simulink model "Ass_3_2024a"  (R2024a)
settings: Solver=VariableStepAuto  StartTime=0.0  StopTime=inf  RelTol=1e-3
model workspace (MAT data in the model file):
  SL_ROS_VariableLengthArrays_MaxSizes.CommonInfo.ArrayTruncateAction = 'EmitWarning'
  SL_ROS_VariableLengthArrays_MaxSizes.MsgTypeMap = containers.Map
  SL_ROS_VariableLengthArrays_MaxSizes.MsgTypeMap.serialization.keys = {'sensor_msgs/Image'}
  SL_ROS_VariableLengthArrays_MaxSizes.MsgTypeMap.serialization.values{1}(1).PropertyName = 'Data'
  SL_ROS_VariableLengthArrays_MaxSizes.MsgTypeMap.serialization.values{1}(1).DataType = 'uint8'
  SL_ROS_VariableLengthArrays_MaxSizes.MsgTypeMap.serialization.values{1}(1).MaxLength = 921600
  SL_ROS_VariableLengthArrays_MaxSizes.MsgTypeMap.serialization.values{1}(2).PropertyName = 'Encoding'
  SL_ROS_VariableLengthArrays_MaxSizes.MsgTypeMap.serialization.values{1}(2).DataType = 'uint8'
  SL_ROS_VariableLengthArrays_MaxSizes.MsgTypeMap.serialization.values{1}(2).MaxLength = 128
  SL_ROS_VariableLengthArrays_MaxSizes.MsgTypeMap.serialization.uniformity = 0
  SL_ROS_VariableLengthArrays_MaxSizes.MsgTypeMap.serialization.keyType = 'char'
  SL_ROS_VariableLengthArrays_MaxSizes.MsgTypeMap.serialization.valueType = 'any'
undefined symbols (not defined in the file or in its folder): Angular, gray, Linear, Rec, SDTV
libraries: robotlib x4, simulink x2, visionstatistics x1, visionconversions x1
settings Model: Creator=daniele

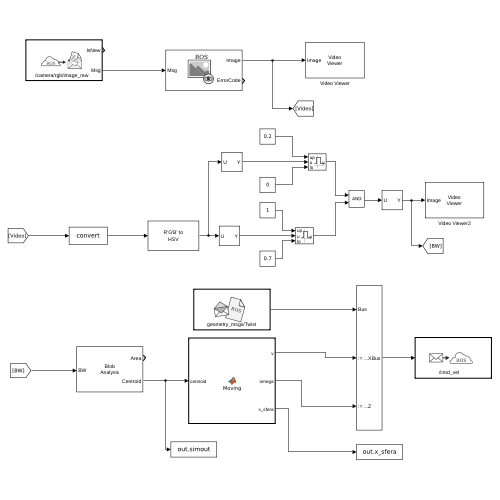
[thumbnail: Simulink's stored preview of the top-level diagram]
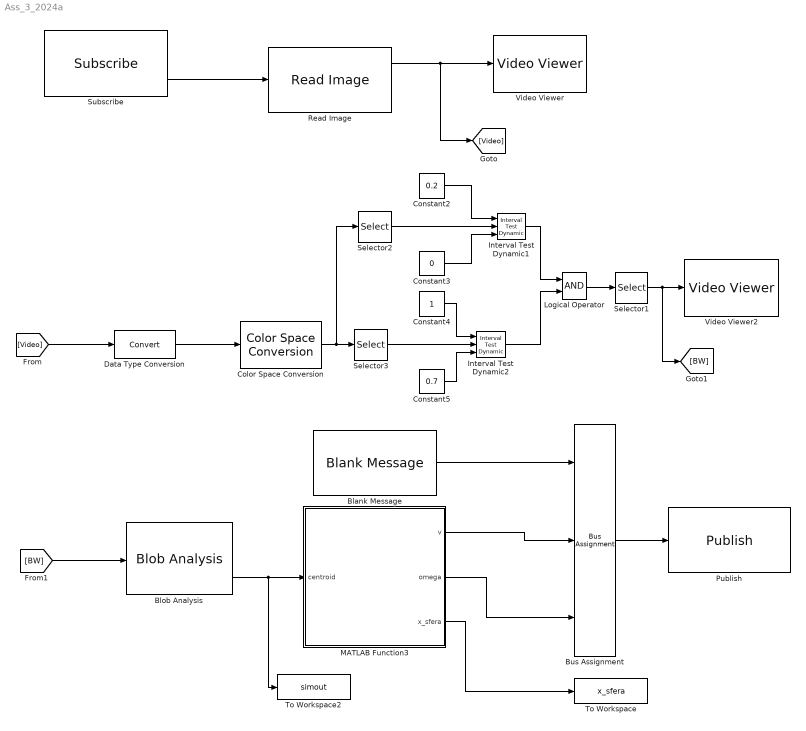
== system Ass_3_2024a ==
  Blank Message : robotlib/Blank Message  messageClass=Message  entityType=geometry_msgs/Twist  messageType=geometry_msgs/Twist  SampleTime=inf  legacyBusStruct=off
  Blob Analysis : visionstatistics/Blob Analysis  Tag=vipblks_row_conv  area=on  centroid=on  bBox=off  majorAxis=off  minorAxis=off  angle=off  eccentricity=off  equivDiameterSq=off  extent=off  perimeter=off  outDT=double  conn=8  isLabel=off  maxBlobs=2  warnIfNumBlobsExceeded=on  isCount=off  useMinArea=off  minArea=0  useMaxArea=off  maxArea=intmax('uint32')  excludeBorderBlob=off  isOutVarDim=off  isFill=on  fillValues=-1  roundingMode=Floor  overflowMode=off  prodOutputMode=Binary point scaling  prodOutputWordLength=32  prodOutputFracLength=16  accumMode=Binary point scaling  accumWordLength=32  accumFracLength=0  outputMode=Binary point scaling  outputWordLength=32  outputFracLength=16  firstCoeffMode=Binary point scaling  firstCoeffWordLength=16  firstCoeffFracLength=14  secondCoeffMode=Binary point scaling  secondCoeffWordLength=32  secondCoeffFracLength=16
  Bus Assignment : BusAssignment  AssignedSignals=Linear.X,Angular.Z
  Color Space Conversion : visionconversions/Color Space  Conversion  conversion=Obsolete  conversionActive=R'G'B' to HSV  wp_str=D65  rec=Rec. 601 (SDTV)  sys=1125/60/2:1  imagePorts=One multidimensional signal
  Constant2 : Constant  Value=0.2
  Constant3 : Constant  Value=0
  Constant4 : Constant
  Constant5 : Constant  Value=0.7
  Data Type Conversion : DataTypeConversion  SaturateOnIntegerOverflow=off  RndMeth=Floor
  Interval Test Dynamic1 : simulink/Logic and Bit Operations/Interval Test Dynamic  IntervalClosedRight=on  IntervalClosedLeft=on  OutDataTypeStr=boolean
  Interval Test Dynamic2 : simulink/Logic and Bit Operations/Interval Test Dynamic  IntervalClosedRight=on  IntervalClosedLeft=on  OutDataTypeStr=boolean
  Logical Operator : Logic  AllPortsSameDT=off  OutDataTypeStr=boolean
  MATLAB Function3 : MATLAB Function  TreatAsAtomicUnit=on
  Publish : robotlib/Publish  topicSource=Select from ROS network  topic=/cmd_vel  messageType=geometry_msgs/Twist  legacyBusStruct=off  messageQueueLength=1
  Read Image : robotlib/Read Image  MaximumImageSize=[480, 640]  ImageEncoding=rgb8  ShowAlphaOutput=off  ShowErrorCodeOutput=on  VariableSizeOutputs=off
  Selector1 : Selector  NumberOfDimensions=2  InputPortWidth=3  IndexOptions=Index vector (dialog),Index vector (dialog)  Indices=[1:480],[1:640]  OutputSizes=1,1
  Selector2 : Selector  NumberOfDimensions=3  InputPortWidth=3  IndexOptions=Index vector (dialog),Index vector (dialog),Index vector (dialog)  Indices=[1:480],[1:640],1  OutputSizes=1,1,1
  Selector3 : Selector  NumberOfDimensions=3  InputPortWidth=3  IndexOptions=Index vector (dialog),Index vector (dialog),Index vector (dialog)  Indices=[1:480],[1:640],2  OutputSizes=1,1,1
  Subscribe : robotlib/Subscribe  topicSource=Select from ROS network  topic=/camera/rgb/image_raw  messageType=sensor_msgs/Image  SampleTime=-1  legacyBusStruct=off  messageQueueLength=1
  To Workspace : ToWorkspace  VariableName=x_sfera  SaveFormat=Timeseries  SampleTime=-1
  To Workspace2 : ToWorkspace  VariableName=simout  SampleTime=-1
  Video Viewer : VideoViewer  colormapValue=gray(256)  FigPos=[73 1078 1828 933]
  Video Viewer2 : VideoViewer  colormapValue=gray(256)  FigPos=[73 1078 1818 933]
  wires:
  Read Image/1 -> [Video], Video Viewer/1
  [Video] -> Data Type Conversion/1
  Subscribe/2 -> Read Image/1
  Constant2/1 -> Interval Test Dynamic1/1
  Constant3/1 -> Interval Test Dynamic1/3
  Constant4/1 -> Interval Test Dynamic2/1
  Constant5/1 -> Interval Test Dynamic2/3
  Logical Operator/1 -> Selector1/1
  Selector1/1 -> [BW], Video Viewer2/1
  Data Type Conversion/1 -> Color Space Conversion/1
  Interval Test Dynamic1/1 -> Logical Operator/1
  Interval Test Dynamic2/1 -> Logical Operator/2
  Color Space Conversion/1 -> Selector2/1, Selector3/1
  Selector2/1 -> Interval Test Dynamic1/2
  Selector3/1 -> Interval Test Dynamic2/2
  MATLAB Function3/1(v) -> Bus Assignment/2
  Blob Analysis/2 -> To Workspace2/1, MATLAB Function3/1(centroid)
  MATLAB Function3/2(omega) -> Bus Assignment/3
  Blank Message/1 -> Bus Assignment/1
  Bus Assignment/1 -> Publish/1
  [BW] -> Blob Analysis/1
  MATLAB Function3/3(x_sfera) -> To Workspace/1

== matlab function Ass_3_2024a/MATLAB Function3 ==
  data: centroid input; v output double; omega output double; x_sfera output

function [v, omega,x_sfera] = Moving(centroid)
    % Parametri della telecamera
    x_img = 320.5;     % Centro dell'immagine in pixel (asse x)
    y_img = 240.5;     % Centro dell'immagine in pixel (asse y)

    % Parametri di controllo
    Kp_angular = 0.002; % Guadagno proporzionale per la velocità angolare (più basso)
    Kp_linear = 0.1;    % Guadagno proporzionale per la velocità lineare
    angular_dead_zone = 15; % Zona morta in pixel per errore angolare
    max_omega = 0.3;    % Velocità angolare massima
    max_v = 0.5;        % Velocità lineare massima

    % Estrai il centroide corretto dai dati
    x_sfera = double(centroid(1)); % Coordinata x del centroide
    y_sfera = double(centroid(2)); % Coordinata y del centroide

    % Errore angolare rispetto al centro dell'immagine
    error_angular = x_sfera - x_img;

    % Zona morta per l'errore angolare
    if abs(error_angular) < angular_dead_zone
        error_angular = 0; % Considera l'errore nullo se è entro la zona morta
    end

    % Smorzamento dell'errore angolare (filtro a media semplice)
    persistent prev_error_angular
    if isempty(prev_error_angular)
        prev_error_angular = error_angular;
    end
    error_angular = 0.7 * prev_error_angular + 0.3 * error_angular;
    prev_error_angular = error_angular;

    % Controllo proporzionale per la velocità angolare
    omega = -Kp_angular * error_angular;

    % Controllo proporzionale per la velocità lineare
    if error_angular == 0
        % Procedi alla massima velocità se la pallina è centrata
        v = max_v;
    else
        % Avanza più lentamente se devi correggere l'angolo
        v = max_v * (1 - min(abs(error_angular) / (x_img / 2), 1));
    end

    % Saturazione delle velocità
    omega = max(min(omega, max_omega), -max_omega);
    v = max(min(v, max_v), 0);

    % Fermo il robot se la pallina non è visibile
    if isnan(x_sfera) || isnan(y_sfera)
        v = 0;
        omega = 0;
    end
end
